simulink model "QiMotorController_ModelReference"  (R2021b)
settings: Solver=FixedStepDiscrete  StartTime=0.0  StopTime=5  RelTol=1e-3
PreLoadFcn:
  | RTWConfigurationCB('preloadfcn', bdroot);
PostLoadFcn:
  | load('configuration/data_struct.mat');
  | load('configuration/fluxMaps_propMotor.mat');
  | load('configuration/parameterInit_PROP.mat');
  | load('configuration/parameterInit_PUMP.mat');
  | load('configuration/parameterInit_PITCH.mat');
  | load('configuration/parameterInit_TILT.mat');
  | %load('configuration/base_workspace_signal_definition.mat');
  | %load('resolvedatastores_to_baseworkspace_for_faster_simulation.mat');
model workspace (MAT data in the model file):
  ADC_CALIBRATION_SAMPLES = Simulink.Parameter
  ADC_CALIBRATION_SAMPLES.Value = 20000
  ADC_CALIBRATION_SAMPLES.Description = 'Number of samples taken by the ADC offset/calibration 
    | function to calibrate the ADC values. Units are in number of 80kHz
    | control interrupts. The time taken to complete the calibration will be
    | equal to:
    | 
    | ADC_CALIBRATION_SAMPLES / (INVERTER_PWM_RATE * 2) seconds
    | '
  ADC_CALIBRATION_SAMPLES.DataType = 'uint32'
  ADC_CALIBRATION_SAMPLES.Complexity = 'real'
  ADC_CALIBRATION_SAMPLES.Dimensions = [1 1]
  DEFAULT_RESOLVER_CONTROL_WORD = Simulink.Parameter
  DEFAULT_RESOLVER_CONTROL_WORD.Value = 97
  DEFAULT_RESOLVER_CONTROL_WORD.DataType = 'uint32'
  DEFAULT_RESOLVER_CONTROL_WORD.Complexity = 'real'
  DEFAULT_RESOLVER_CONTROL_WORD.Dimensions = [1 1]
  PLL_FREQUENCY = Simulink.Parameter
  PLL_FREQUENCY.Value = 100000000
  PLL_FREQUENCY.Description = '100 MHz'
  PLL_FREQUENCY.DataType = 'double'
  PLL_FREQUENCY.Complexity = 'real'
  PLL_FREQUENCY.Dimensions = [1 1]
  SIMULATION_OPTIONS = Simulink.Parameter
  SIMULATION_OPTIONS.Value = 0
  SIMULATION_OPTIONS.Description = 'Set to ''0'' for normal Simulation
    | Set to ''1'' for "Flying Start" simulation'
  SIMULATION_OPTIONS.DataType = 'uint32'
  SIMULATION_OPTIONS.Complexity = 'real'
  SIMULATION_OPTIONS.Dimensions = [1 1]
  TARGET_CODE_GEN = Simulink.Parameter
  TARGET_CODE_GEN.Value = 0
  TARGET_CODE_GEN.Description = 'Set to ''0'' for Plant Model or PIL Simulation
    | Set to ''1'' for Target System Code Generation'
  TARGET_CODE_GEN.DataType = 'uint32'
  TARGET_CODE_GEN.Complexity = 'real'
  TARGET_CODE_GEN.Dimensions = [1 1]
  Ts = 2.5e-07
undefined symbols (not defined in the file): DEADTIME_NS__PITCH, DEADTIME_NS__PROP, DEADTIME_NS__PUMP, DEADTIME_NS__TILT, fIa_, fIb_, fIc_, fIdc_, fMotorEncoderFloat_, fMotorSensorSpeed_, fUa_, fUb_, fUc_, fUdc_, inbtilt, mdl_pitch_uiAPUFlags, mdl_pitch_uiFlags, modelData, oMot_, oOut_, opInputResolverData_, oPitch, oState_, PLANT_SPEED_QUADRATIC_COEFF__PUMP, POLE_PAIRS_INIT__PITCH, POLE_PAIRS_INIT__PROP, POLE_PAIRS_INIT__PUMP, POLE_PAIRS_INIT__TILT, PWM_FREQ_KHZ__PITCH, PWM_FREQ_KHZ__PROP, PWM_FREQ_KHZ__PUMP, R_PHASE_INIT__PITCH, R_PHASE_INIT__PROP, R_PHASE_INIT__TILT, R_PHASE_INIT_PLANT__PUMP, uiControlReadback_, uiGateDriverStatus_
libraries: simulink x51, spsSeriesRLCBranchLib x25, spsMosfetLib x24, powerlib_extras x24, spsCurrentMeasurementLib x17, spsVoltageMeasurementLib x17, spsPermanentMagnetSynchronousMachineLib x3, spsDCVoltageSourceLib x2, motorModelLibrary x2, slpidlib x2, cstblocks x1, spspowerguiLib x1
(part 1 of 5)
Description:
  | /************************************************************
  | /* (c) 2013 Phasor Systems, Incorporated
  | /* All rights reserved
  | /*
  | /* Model provided under End User License Agreement or OEM License Agreement
  | /*
  | /* Use of this model is your acceptance of the terms and conditions of these
  | /* agreements.
  | /*
  | /************************************************************
settings Model: ModifiedComment=Brad -- Sat Feb 01 15:53:39 2014 -- Version 1.11  Creator=Brad Landseadel  LastModifiedBy=jessica.colton
settings Model: ModifiedHistory=|
  | Brad -- Sat Feb 01 15:53:39 2014 -- Version 1.11
  | 
  | 
  | Brad -- Sat Feb 01 15:53:39 2014 -- Version 1.11
  | 
  | 
  | Brad -- Sat Feb 01 15:48:49 2014 -- Version 1.10
  | 
  | 
  | Brad -- Sat Feb 01 15:38:18 2014 -- Version 1.9
  | 
  | 
  | Brad -- Sat Feb 01 15:22:57 2014 -- Version 1.8
  | 
  | 
  | Brad -- Sat Feb 01 15:08:45 2014 -- Version 1.7
  | 
  | 
  | Brad -- Sat Feb 01 14:46:18 2014 -- Version 1.6
  | 
  | 
  | Brad -- Sat Feb 01 13:34:06 2014 -- Version 1.5
  | 
  | 
  | Brad -- Sat Feb 01 13:29:08 2014 -- Version 1.4
  | 
  | 
  | Brad -- Sat Feb 01 13:18:41 2014 -- Version 1.3
  | 
  | 
  | Brad -- Sat Feb 01 12:30:13 2014 -- Version 1.2
settings SolverCC: AlgebraicLoopSolver=TrustRegion  PositivePriorityOrder=on
settings DataIOCC: LimitDataPoints=on  SaveFormat=Array  SignalLoggingSaveFormat=ModelDataLogs  SaveOutput=off  SaveTime=off  ReturnWorkspaceOutputs=off
settings OptimizationCC: DefaultParameterBehavior=Inlined  GainParamInheritBuiltInType=on  UseFloatMulNetSlope=on  DefaultUnderspecifiedDataType=single  InlineInvariantSignals=on  StrengthReduction=on  PassReuseOutputArgsAs=Individual arguments  ExpressionDepthLimit=2147483647  ZeroExternalMemoryAtStartup=off  ZeroInternalMemoryAtStartup=off  NoFixptDivByZeroProtection=on  EfficientFloat2IntCast=on  MaxStackSize=2000  SimCompilerOptimization=on  AccelVerboseBuild=on  OptimizeBlockOrder=speed  UseRowMajorAlgorithm=on  OptimizationPriority=Speed  LabelGuidedReuse=on  MultiThreadedLoops=on  EfficientTunableParamExpr=on
settings DebuggingCC: ReadBeforeWriteMsg=DisableAll  WriteAfterReadMsg=DisableAll  MergeDetectMultiDrivingBlocksExec=none  SolverPrmCheckMsg=warning  MultiTaskDSMMsg=none  MultiTaskRateTransMsg=warning  ParameterTunabilityLossMsg=error  FixptConstUnderflowMsg=error  FixptConstOverflowMsg=error  BusObjectLabelMismatch=error  AssertControl=DisableAll  AllowSymbolicDim=off  StateNameClashWarn=warning  SFUnexpectedBacktrackingDiag=warning  SFNoUnconditionalDefaultTransitionDiag=warning  SFExecutionAtInitializationDiag=none  SFMachineParentedDataDiag=warning  ArithmeticOperatorsInVariantConditions=warning
settings HardwareCC: ProdBitPerPointer=32  ProdBitPerSizeT=32  ProdBitPerPtrDiffT=32  ProdLargestAtomicInteger=Long  ProdLargestAtomicFloat=Double  ProdWordSize=32  ProdHWDeviceType=ARM Compatible->ARM Cortex-A  TargetLargestAtomicInteger=Long  TargetLargestAtomicFloat=Double  TargetIntDivRoundTo=Zero  TargetEndianess=LittleEndian  TargetHWDeviceType=ARM Compatible->ARM Cortex-A
settings ModelReferenceCC: UpdateModelReferenceTargets=IfOutOfDate  PropagateSignalLabelsOutOfModel=off
settings SFSimCC: SimCustomHeaderCode="//#include \"custom_code/second_level_include/math_special.h\""  SimUserSources=//math_special.c  SimUserIncludeDirs=//custom_code/src/  SFSimEcho=off  SimUseLocalCustomCode=off  MATLABDynamicMemAlloc=off  CustomCodeUndefinedFunction=UseInterfaceOnly
settings RTWCC: Description=Embedded Coder  SystemTargetFile=ert.tlc  GenCodeOnly=on  PackageGeneratedCodeAndArtifacts=on  TemplateMakefile=ert_default_tmf  GenerateReport=on  RetainRTWFile=on  RTWUseLocalCustomCode=off  CustomSource=custom_code/src/math_special.c  Toolchain=GNU gcc/g++ | gmake (64-bit Linux)  BuildConfiguration=Faster Runs  IncludeHyperlinkInReport=on  LaunchReport=on  GenerateTraceInfo=on  GenerateTraceReport=on  GenerateTraceReportSl=on  GenerateTraceReportSf=on  GenerateTraceReportEml=on  GenerateWebview=on  GenerateCodeMetricsReport=on  GenerateCodeReplacementReport=on  CheckMdlBeforeBuild=Warning
settings RTWCC: CustomHeaderCode=|
  | #include "../custom_code/second_level_include/math_special.h"
  | 
  | // FPGA interface
  | #include "../custom_code/include/motorTask_int.h"
  | #include "../custom_code/include/motorControl_common.h"
  | #include "../custom_code/include/common.h"
  | #include "../custom_code/include/motorControl_adc.h"
  | #include "../custom_code/include/motorControl_pwm.h"
  | 
  | // InterCore
  | #include "../custom_code/inverter_shared_memory/legacy_inverter_shared_memory_declaration.h"
  | 
  | // Second Level Includes
  | #include "../custom_code/second_level_include/adc.h"
  | #include "../custom_code/second_level_include/application_layer_com.h"
  | #include "../custom_code/second_level_include/gate_enable.h"
  | #include "../custom_code/second_level_include/housekeeping.h"
  | #include "../custom_code/second_level_include/hw_defines.h"
  | #include "../custom_code/second_level_include/iir.h"
  | #include "../custom_code/second_level_include/legacy_interCoreCom.h"
  | #include "../custom_code/second_level_include/motor_control_main.h"
  | #include "../custom_code/second_level_include/motorControl_common.h"
  | #include "../custom_code/second_level_include/motorTask_init.h"
  | #include "../custom_code/second_level_include/motorTask_intercoreCom.h"
  | #include "../custom_code/second_level_include/motorTask_main.h"
  | #include "../custom_code/second_level_include/motorTask_StateMachine.h"
  | #include "../custom_code/second_level_include/parameter_init.h"
  | #include "../custom_code/second_level_include/pattern_generator.h"
  | #include "../custom_code/second_level_include/pi_controller.h"
  | #include "../custom_code/second_level_include/platform.h"
  | #include "../custom_code/second_level_include/pwm.h"
  | #include "../custom_code/second_level_include/resolver_driver.h"
  | #include "../custom_code/second_level_include/software_identity_data_storage.h"
  | #include "../custom_code/second_level_include/std_math.h"
settings CodeAppCC: ForceParamTrailComments=on  IgnoreCustomStorageClasses=off  IgnoreTestpoints=on  MaxIdLength=128  OperatorAnnotations=on  SimulinkDataObjDesc=on  SFDataObjDesc=on  InsertBlockDesc=on  StateflowObjectComments=on
settings ERTTargetCC: TargetLangStandard=C99 (ISO)  CombineSignalStateStructs=on  GroupInternalDataByFunction=on  SuppressErrorStatus=on  SupportComplex=off  ParenthesesLevel=Maximum  CastingMode=Explicit  RootIOFormat=Structure reference  ERTCustomFileTemplate=example_file_process.tlc
settings ConfigComp: CovMetricSettings=dw  CovSaveCumulativeToWorkspaceVar=on  CovSaveSingleToWorkspaceVar=on  CovExternalEMLEnable=off  CovSFcnEnable=off
settings SimscapeCC: SimscapeNormalizeSystem=off

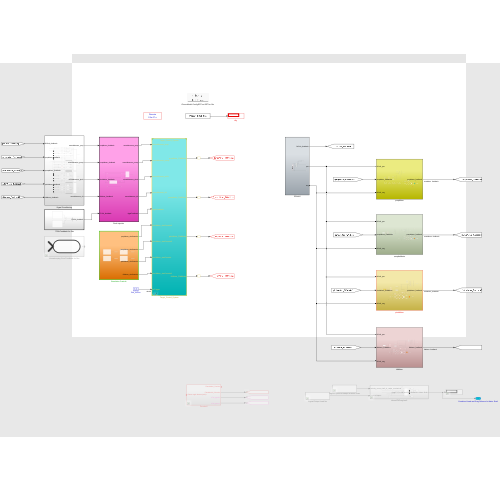
[thumbnail: Simulink's stored preview of the top-level diagram]
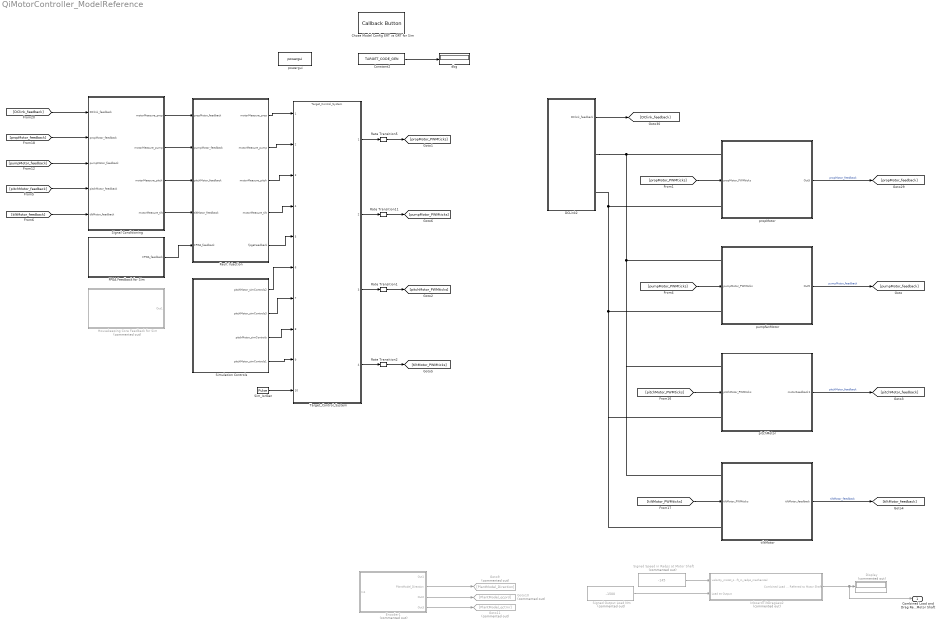
== system QiMotorController_ModelReference ==
  Chose Model Config ERT vs GRT for Sim : CallbackButton  ButtonText=Chose ERT vs GRT for Sim
      settings: ClickFcn=|
      | TARGET_CODE_GEN_LOCAL = getVariable( get_param('PMSM_Sensorless_Propulsion_Model_Code_Generation_Struct','ModelWorkspace'),'TARGET_CODE_GEN').Value;
      | 
      | if( TARGET_CODE_GEN_LOCAL == 0 )
      |  setActiveConfigSet('PMSM_Sensorless_Propulsion_Model_Code_Generation_Struct', 'grt_simulated_config');
      |  get_param(getActiveConfigSet('PMSM_Sensorless_Propulsion_Model_Code_Generation_Struct'),'Name')
      | end
      | 
      | if( TARGET_CODE_GEN_LOCAL == 1 )
      |  setActiveConfigSet('PMSM_Sensorless_Propulsion_Model_Code_Generation_Struct', 'Xilinx_Zynq_Core4');
      |  get_param(getActiveConfigSet('PMSM_Sensorless_Propulsion_Model_Code_Generation_Struct'),'Name')
      | end
  Constant2 : Constant  Value=TARGET_CODE_GEN  OutDataTypeStr=boolean  SampleTime=-1
  DCLink2 : Subsystem
  Display : Display  Commented=on
  Encoder1 : Subsystem  Commented=on
  FPGA Feedback for Sim : Subsystem  TreatAsAtomicUnit=on  SystemSampleTime=1/(PWM_FREQ_KHZ__PROP*1000)/2
  Fault Injection : Subsystem  TreatAsAtomicUnit=on  SystemSampleTime=1/(PWM_FREQ_KHZ__PROP*1000)/2
  Goto10 : Goto  Commented=on  GotoTag=PlantModel_qcprd
  Goto11 : Goto  Commented=on  GotoTag=PlantModel_qctmr
  Goto9 : Goto  Commented=on  GotoTag=PlantModel_Direction
  Housekeeping Core Feedback for Sim : Subsystem  Commented=on
  InboardTiltDragLaw2 : Subsystem  Commented=on
  Rate Transition{1..2,5,11} (4 alike) : RateTransition  Deterministic=off  OutPortSampleTime=Ts
  Signal Conditioning : Subsystem
  Signed Output Load Nm : Constant  Commented=on  Value=-1500  OutDataTypeStr=single  SampleTime=1e-2
  Signed Speed in Radps at Motor Shaft : Constant  Commented=on  Value=-145  OutDataTypeStr=single  SampleTime=1e-2
  Sim_IsrGen : DiscretePulseGenerator  PulseType=Time based  Period=1/(PWM_FREQ_KHZ__PROP*1000)/2  PulseWidth=50
  Simulation Controls : Subsystem  TreatAsAtomicUnit=on  SystemSampleTime=1/(PWM_FREQ_KHZ__PROP*1000)/2
  Target_Control_System : ModelReference  ModelNameDialog=Target_Control_System  SimulationMode=Normal  ModelReferenceVersion=4.101
  dbg : Display
      settings: Format=decimal (Stored Integer)
  pitchMotor : Subsystem
      settings: PortSchema="{\"entries\":[{\"content\":{\"sides\":[{\"content\":{\"connectorIds\":[\"LConn1\",\"In1\",\"LConn2\"]},\"type\":\"ConnectorPlacement.EquallySpacedRectSide\",\"uuid\":\"2948c356-2dfc-4425-a4d7-a3951926bd60\"},{\"content\":{\"connectorIds\":[\"Out1\"],\"side\":\"RIGHT\"},\"type\":\"ConnectorPlacement.EquallySpacedRectSide\",\"uuid\":\"906a8e9a-2635-4c14-9d40-34f0713bab39\"},{\"content\":{\"connectorIds\":[],\"side\":\"TOP\"},\"type\":\"ConnectorPlacement.EquallySpacedRectSide\",\"uuid\":\"336ec430-6931-46f0-bbde-94f235c37a61\"},{\"content\":{\"connectorIds\":[],\"side\":\"HIDDEN\"},\"type\":\"ConnectorPlacement.EquallySpacedRectSide\",\"uuid\":\"b760127f-7c64-4918-bd3a-cb813c8c851d\"}]},\"type\":\"ConnectorPlacement.EquallySpacedConnector\",\"uuid\":\"386eabba-acb8-4870-b3f4-1d48c2148e04\"}],\"packageUris\":[\"http://schema.mathworks.com/mf0/Connector/R2020b\"],\"version\":\"1.0\"}"
  powergui : spspowerguiLib/powergui  SimulationMode=Discrete  SampleTime=Ts  frequency=60  Iterations=50  frequencyindice=0  Pbase=100e6  ErrMax=1e-4  UnitsV=kV  UnitsW=MW  buscounter=0  FunctionMessages=off  echomessages=off  EnableUseOfTLC=off  CurrentSourceSwitches=off  DisableSnubberDevices=off  DisableRonSwitches=off  DisableVfSwitches=off  DisplayEquations=off  AutomaticDiscreteSolvers=off  SolverType=Tustin  Interpol=off  ExternalGateDelay=off  methode=off  Ts=0  x0status=blocks  SPID=off  SwTol=0  HookPort=off  NonlinearTolerance=1e-4  nMaxIteration=100  ContinueOnMaxIteration=off  RestoreLinks=warning  ResistiveCurrentMeasurement=off  Frange=[0:2:500]  Ylog=off  Xlog=on  ShowGrid=off  save=off  variable=ZData  structure=0  ZoomFFT=on  StartTime=0.0  cycles=1  DisplayStyle=1  fundamental=60  FreqAxis=off  MaxFrequency=1000  frequencyindicesteady=1  RmsSteady=1  display=off
  propMotor : Subsystem
      settings: PortSchema="{\"entries\":[{\"content\":{\"sides\":[{\"content\":{\"connectorIds\":[\"LConn1\",\"In1\",\"LConn2\"]},\"type\":\"ConnectorPlacement.EquallySpacedRectSide\",\"uuid\":\"2948c356-2dfc-4425-a4d7-a3951926bd60\"},{\"content\":{\"connectorIds\":[\"Out1\"],\"side\":\"RIGHT\"},\"type\":\"ConnectorPlacement.EquallySpacedRectSide\",\"uuid\":\"906a8e9a-2635-4c14-9d40-34f0713bab39\"},{\"content\":{\"connectorIds\":[],\"side\":\"TOP\"},\"type\":\"ConnectorPlacement.EquallySpacedRectSide\",\"uuid\":\"336ec430-6931-46f0-bbde-94f235c37a61\"},{\"content\":{\"connectorIds\":[],\"side\":\"HIDDEN\"},\"type\":\"ConnectorPlacement.EquallySpacedRectSide\",\"uuid\":\"b760127f-7c64-4918-bd3a-cb813c8c851d\"}]},\"type\":\"ConnectorPlacement.EquallySpacedConnector\",\"uuid\":\"386eabba-acb8-4870-b3f4-1d48c2148e04\"}],\"packageUris\":[\"http://schema.mathworks.com/mf0/Connector/R2020b\"],\"version\":\"1.0\"}"
  pumpfanMotor : Subsystem
      settings: PortSchema="{\"entries\":[{\"content\":{\"sides\":[{\"content\":{\"connectorIds\":[\"LConn1\",\"In1\",\"LConn2\"]},\"type\":\"ConnectorPlacement.EquallySpacedRectSide\",\"uuid\":\"2948c356-2dfc-4425-a4d7-a3951926bd60\"},{\"content\":{\"connectorIds\":[\"Out1\"],\"side\":\"RIGHT\"},\"type\":\"ConnectorPlacement.EquallySpacedRectSide\",\"uuid\":\"906a8e9a-2635-4c14-9d40-34f0713bab39\"},{\"content\":{\"connectorIds\":[],\"side\":\"TOP\"},\"type\":\"ConnectorPlacement.EquallySpacedRectSide\",\"uuid\":\"336ec430-6931-46f0-bbde-94f235c37a61\"},{\"content\":{\"connectorIds\":[],\"side\":\"HIDDEN\"},\"type\":\"ConnectorPlacement.EquallySpacedRectSide\",\"uuid\":\"b760127f-7c64-4918-bd3a-cb813c8c851d\"}]},\"type\":\"ConnectorPlacement.EquallySpacedConnector\",\"uuid\":\"386eabba-acb8-4870-b3f4-1d48c2148e04\"}],\"packageUris\":[\"http://schema.mathworks.com/mf0/Connector/R2020b\"],\"version\":\"1.0\"}"
  tiltMotor : Subsystem
      settings: PortSchema="{\"entries\":[{\"content\":{\"sides\":[{\"content\":{\"connectorIds\":[\"LConn1\",\"In1\",\"LConn2\"]},\"type\":\"ConnectorPlacement.EquallySpacedRectSide\",\"uuid\":\"2948c356-2dfc-4425-a4d7-a3951926bd60\"},{\"content\":{\"connectorIds\":[\"Out1\"],\"side\":\"RIGHT\"},\"type\":\"ConnectorPlacement.EquallySpacedRectSide\",\"uuid\":\"906a8e9a-2635-4c14-9d40-34f0713bab39\"},{\"content\":{\"connectorIds\":[],\"side\":\"TOP\"},\"type\":\"ConnectorPlacement.EquallySpacedRectSide\",\"uuid\":\"336ec430-6931-46f0-bbde-94f235c37a61\"},{\"content\":{\"connectorIds\":[],\"side\":\"HIDDEN\"},\"type\":\"ConnectorPlacement.EquallySpacedRectSide\",\"uuid\":\"b760127f-7c64-4918-bd3a-cb813c8c851d\"}]},\"type\":\"ConnectorPlacement.EquallySpacedConnector\",\"uuid\":\"386eabba-acb8-4870-b3f4-1d48c2148e04\"}],\"packageUris\":[\"http://schema.mathworks.com/mf0/Connector/R2020b\"],\"version\":\"1.0\"}"
  Combined Load and Drag Referred to Motor Shaft : Outport
  wires:
  Rate Transition5/1 -> [propMotor_PWMticks]
  Encoder1/2(PlantModel_Direction) -> Goto9/1
  Encoder1/3(Out2) -> Goto10/1
  Encoder1/4(Out3) -> Goto11/1
  Constant2/1 -> dbg/1
  [propMotor_PWMticks] -> propMotor/1(propMotor_PWMticks)
  DCLink2/1(DClink_feedback) -> [DClink_feedback]
  propMotor/1(Out5) -> [propMotor_feedback]  "propMotor_feedback"
  pumpfanMotor/1(Out5) -> [pumpMotor_feedback]  "pumpMotor_feedback"
  [pitchMotor_PWMticks] -> pitchMotor/1(pitchMotor_PWMticks)
  [tiltMotor_PWMticks] -> tiltMotor/1(tiltMotor_PWMticks)
  [pumpMotor_feedback] -> Signal Conditioning/3(pumpMotor_feedback)
  [propMotor_feedback] -> Signal Conditioning/2(propMotor_feedback)
  [DClink_feedback] -> Signal Conditioning/1(DClink_feedback)
  pitchMotor/1(motorFeedback1) -> [pitchMotor_feedback]  "pitchMotor_feedback"
  tiltMotor/1(tiltMotor_feedback) -> [tiltMotor_feedback]  "tiltMotor_feedback"
  [pumpMotor_PWMticks] -> pumpfanMotor/1(pumpMotor_PWMticks)
  [tiltMotor_feedback] -> Signal Conditioning/5(tiltMotor_feedback)
  [pitchMotor_feedback] -> Signal Conditioning/4(pitchMotor_feedback)
  Signal Conditioning/1(motorMeasure_prop) -> Fault Injection/1(propMotor_feedback)
  Signal Conditioning/2(motorMeasure_pump) -> Fault Injection/2(pumpMotor_feedback)
  Signal Conditioning/4(motorMeasure_tilt) -> Fault Injection/4(tiltMotor_feedback)
  Signal Conditioning/3(motorMeasure_pitch) -> Fault Injection/3(pitchMotor_feedback)
  Target_Control_System/2 -> Rate Transition11/1
  Rate Transition11/1 -> [pumpMotor_PWMticks]
  Target_Control_System/1 -> Rate Transition5/1
  Target_Control_System/3 -> Rate Transition1/1
  Rate Transition1/1 -> [pitchMotor_PWMticks]
  Signed Output Load Nm/1 -> InboardTiltDragLaw2/2(Load at Output)
  InboardTiltDragLaw2/1(Combined Load and Drag Referred to Motor Shaft) -> Display/1, Combined Load and Drag Referred to Motor Shaft/1
  Signed Speed in Radps at Motor Shaft/1 -> InboardTiltDragLaw2/1(velocity_motot_shaft_in_radps_mechanical)
  Rate Transition2/1 -> [tiltMotor_PWMticks]
  Target_Control_System/4 -> Rate Transition2/1
  FPGA Feedback for Sim/1(FPGA_feedback) -> Fault Injection/5(FPGA_feedback)
  Simulation Controls/1(pitchMotor_simControls2) -> Target_Control_System/6
  Simulation Controls/2(pitchMotor_simControls3) -> Target_Control_System/7
  Simulation Controls/3(pitchMotor_simControls) -> Target_Control_System/8
  Simulation Controls/4(pitchMotor_simControls1) -> Target_Control_System/9
  Fault Injection/1(motorMeasure_prop) -> Target_Control_System/1
  Fault Injection/5(fpgaFeedback) -> Target_Control_System/5
  Fault Injection/2(motorMeasure_pump) -> Target_Control_System/2
  Fault Injection/4(motorMeasure_tilt) -> Target_Control_System/4
  Fault Injection/3(motorMeasure_pitch) -> Target_Control_System/3
  Sim_IsrGen/1 -> Target_Control_System/10
  connections:
  DCLink2/RConn1 -- pitchMotor/LConn1 -- tiltMotor/LConn1 -- pumpfanMotor/LConn1 -- propMotor/LConn1
  tiltMotor/LConn2 -- pitchMotor/LConn2 -- pumpfanMotor/LConn2 -- DCLink2/RConn2 -- propMotor/LConn2

== system QiMotorController_ModelReference/DCLink2 ==
  Battery internal resistance2 : spsSeriesRLCBranchLib/Series RLC Branch  LConnTagsString=__new0  RConnTagsString=__new0  BranchType=R  Resistance=0.4  Inductance=33e-9  SetiL0=off  InitialCurrent=0  Capacitance=470e-6  Setx0=off  InitialVoltage=0  Measurements=None
  Bus Creator : BusCreator  Inputs=2
  CT2 : spsCurrentMeasurementLib/Current Measurement  PhasorSimulation=off  OutputType=Complex  PSBequivalent=0
  VDC4 : spsDCVoltageSourceLib/DC Voltage Source  Amplitude=700/2  Measurements=None
  VDC5 : spsDCVoltageSourceLib/DC Voltage Source  Amplitude=700/2  Measurements=None
  VM3 : spsVoltageMeasurementLib/Voltage Measurement  PhasorSimulation=off  OutputType=Complex  PSBequivalent=0
  pos : PMIOPort  Side=Right
  neg : PMIOPort  Port=2  Side=Right
  DClink_feedback : Outport
  wires:
  CT2/1 -> Bus Creator/1  "DClinkCurrent"
  Bus Creator/1 -> DClink_feedback/1  "DClink_feedback"
  VM3/1 -> Bus Creator/2  "DClinkVoltage"
  connections:
  VDC5/RConn1 -- Battery internal resistance2/RConn1
  VM3/LConn2 -- neg/RConn1 -- VDC4/LConn1
  CT2/RConn1 -- pos/RConn1
  VM3/LConn1 -- Battery internal resistance2/LConn1 -- CT2/LConn1
  VDC4/RConn1 -- VDC5/LConn1

== system QiMotorController_ModelReference/Encoder1 ==
  In1 : Inport
  1/T Simulation : Subsystem  Commented=on
  Convert rotor angle to counts : Constant  Value=2*pi/(4095*2)  SampleTime=-1
  Data Type Conversion : DataTypeConversion  OutDataTypeStr=uint16
  Detect Change : simulink/Logic and Bit Operations/Detect Change  Commented=on  vinit=0  OutDataTypeStr=boolean
  Detect Decrease : simulink/Logic and Bit Operations/Detect Decrease  vinit=0.0  OutDataTypeStr=boolean
  Detect Increase : simulink/Logic and Bit Operations/Detect Increase  vinit=0.0  OutDataTypeStr=boolean
  Display3 : Display
  Divide : Product  Inputs=*/  RndMeth=Nearest
  Goto6 : Goto  Commented=on  GotoTag=PM_eCAP_Capture
  Goto8 : Goto  Commented=on  GotoTag=PM_eCAP_TSCounter
  Logical Operator : Logic  IconShape=distinctive  AllPortsSameDT=off  OutDataTypeStr=boolean
  Logical Operator1 : Logic  Operator=NOT  IconShape=distinctive  AllPortsSameDT=off  OutDataTypeStr=boolean
  Math Function : Math  Operator=mod  SignedPower=on  SaturateOnIntegerOverflow=on
  Modulo : Constant  Value=4095*2  SampleTime=-1
  Scope2 : Scope  Commented=on  NumInputPorts=4
  Scope3 : Scope  Commented=on  NumInputPorts=3
  Unary Minus : UnaryMinus
  Out1 : Outport
  PlantModel_Direction : Outport  Port=2
  Out2 : Outport  Port=3
  Out3 : Outport  Port=4
  wires:
  Convert rotor angle to counts/1 -> Divide/2
  Divide/1 -> Math Function/1  "PlantModel_Position"
  Modulo/1 -> Math Function/2
  In1/1 -> Unary Minus/1
  Logical Operator/1 -> Scope2/3, PlantModel_Direction/1  "PlantModel_Direction"
  Detect Increase/1 -> Logical Operator/1
  Detect Decrease/1 -> Logical Operator1/1
  Logical Operator1/1 -> Logical Operator/2
  Unary Minus/1 -> Detect Decrease/1, Detect Increase/1, Scope2/1, Divide/1
  Math Function/1 -> Display3/1, Data Type Conversion/1
  1/T Simulation/1(Out1) -> Scope3/1, Goto6/1, Out2/1
  1/T Simulation/2(Out2) -> Out3/1, Goto8/1, Scope3/2
  Detect Change/1 -> 1/T Simulation/1(In3), Scope3/3
  Data Type Conversion/1 -> Scope2/2, Out1/1, Detect Change/1  "PlantModel_Position"

== system QiMotorController_ModelReference/FPGA Feedback for Sim ==
  Bus Creator2 : BusCreator  Inputs=2
  Rate Transition1 : RateTransition
  Rate Transition11 : RateTransition
  pitchMotor : Subsystem  TreatAsAtomicUnit=on
  tiltMotor : Subsystem  TreatAsAtomicUnit=on
  FPGA_feedback : Outport
  wires:
  pitchMotor/1(Out1) -> Rate Transition11/1  "pitchMotor_FPGAfeedback"
  Rate Transition1/1 -> Bus Creator2/2  "tiltMotor_FPGAfeedback"
  Rate Transition11/1 -> Bus Creator2/1  "pitchMotor_FPGAfeedback"
  tiltMotor/1(Out1) -> Rate Transition1/1  "tiltMotor_FPGAfeedback"
  Bus Creator2/1 -> FPGA_feedback/1

== system QiMotorController_ModelReference/Fault Injection ==
  propMotor_feedback : Inport  OutDataTypeStr=Bus: SAdcDataSingleIn_t
  pumpMotor_feedback : Inport  Port=2  OutDataTypeStr=Bus: SAdcDataSingleIn_t
  pitchMotor_feedback : Inport  Port=3  OutDataTypeStr=Bus: SAdcDataSingleIn_t
  tiltMotor_feedback : Inport  Port=4  OutDataTypeStr=Bus: SAdcDataSingleIn_t
  FPGA_feedback : Inport  Port=5
  Bus Assignment1 : BusAssignment  AssignedSignals=pitchMotor_FPGAfeedback
  Bus Selector : BusSelector  OutputSignals=pitchMotor_FPGAfeedback
  pitchMotor_faults : Subsystem  TreatAsAtomicUnit=on
  motorMeasure_prop : Outport  OutDataTypeStr=Bus: SAdcDataSingleIn_t
  motorMeasure_pump : Outport  Port=2  OutDataTypeStr=Bus: SAdcDataSingleIn_t
  motorMeasure_pitch : Outport  Port=3  OutDataTypeStr=Bus: SAdcDataSingleIn_t
  motorMeasure_tilt : Outport  Port=4  OutDataTypeStr=Bus: SAdcDataSingleIn_t
  fpgaFeedback : Outport  Port=5
  wires:
  propMotor_feedback/1 -> motorMeasure_prop/1
  pumpMotor_feedback/1 -> motorMeasure_pump/1
  tiltMotor_feedback/1 -> motorMeasure_tilt/1
  pitchMotor_feedback/1 -> pitchMotor_faults/1(pitchMotor_feedback)
  pitchMotor_faults/1(motorMeasure_pitch) -> motorMeasure_pitch/1
  FPGA_feedback/1 -> Bus Selector/1, Bus Assignment1/1
  pitchMotor_faults/2(fpgaFeedback_pitch) -> Bus Assignment1/2
  Bus Selector/1 -> pitchMotor_faults/2(pitchMotor_FPGAfeedback)  "<pitchMotor_FPGAfeedback>"
  Bus Assignment1/1 -> fpgaFeedback/1

== system QiMotorController_ModelReference/Housekeeping Core Feedback for Sim ==
  Out1 : Outport

== system QiMotorController_ModelReference/InboardTiltDragLaw2 ==
  velocity_motot_shaft_in_radps_mechanical : Inport
  Load at Output : Inport  Port=2
  DefaultTemp : Constant  Value=45  OutDataTypeStr=single  SampleTime=1e-2
  Display : Display
  Display1 : Display
  Display2 : Display
  DocBlock : simulink/Model-Wide Utilities/DocBlock  DocumentType=Text
      content=|
      | /// \breif Check in what drag mode we are currently running; this is for tilts only
      |    /// Logic table: -1, not floppy; -1 floppy;  use dMechanicalEfficiency_ in the 1st case; in the 2nd, does not matter FD does the calcs
      |    ///               0, not floppy;  0 floppy;  use dMechanicalEfficiency_ only for the 1st of the two
      |    ///               >0, not floppy; >0 floppy;  do not use dMechanicaEfficiency_ in either mode, i.e. set it to 1Type your documentation here
  DocBlock1 : simulink/Model-Wide Utilities/DocBlock  DocumentType=Text
      content=|
      | This is used to make comparison to stick torque when commensing actuator motion.
      | Defaulting to 0 for simplicity. Connect to actual electrical torque as needed for testing
  MotoredOrNot : Constant  OutDataTypeStr=single  SampleTime=1e-2
  SimplifiedVersion : Constant  Value=0  OutDataTypeStr=single  SampleTime=1e-2
  Subsystem1 : Subsystem
  Sum4 : Sum
  WhichDragCalcSeeDoc : Constant  OutDataTypeStr=single  SampleTime=1e-2
  drag2 : Subsystem
  Combined Load and Drag Referred to Motor Shaft : Outport
  wires:
  Subsystem1/1(torque_load_m) -> drag2/4(torque_load_m)
  velocity_motot_shaft_in_radps_mechanical/1 -> drag2/2(velocity_m)
  Sum4/1 -> Combined Load and Drag Referred to Motor Shaft/1, Display2/1
  WhichDragCalcSeeDoc/1 -> drag2/6(DrgMlt), Subsystem1/2(DrgMlt)
  DefaultTemp/1 -> drag2/3(motor_temp)
  SimplifiedVersion/1 -> drag2/1(torque_out_m)
  Load at Output/1 -> Subsystem1/1(torque_load)
  MotoredOrNot/1 -> drag2/5(n_invs), Subsystem1/3(n_inv)
  drag2/1(drag_torque) -> Display/1, Sum4/1
  drag2/2(load_torque) -> Sum4/2, Display1/1

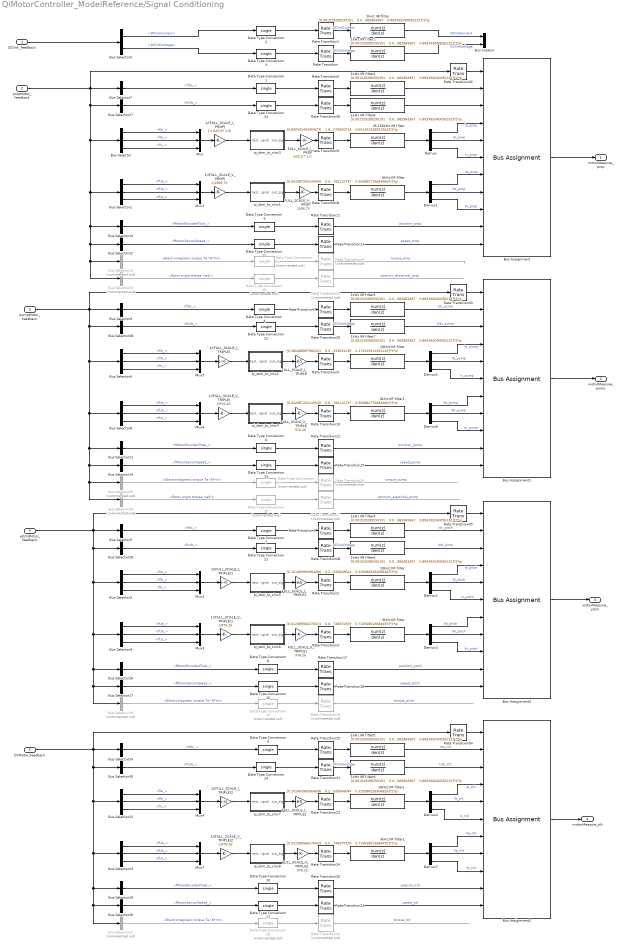
== system QiMotorController_ModelReference/Signal Conditioning ==
  DClink_feedback : Inport
  propMotor_feedback : Inport  Port=2  OutDataTypeStr=Bus: SAdcDataSingleIn_t
  pumpMotor_feedback : Inport  Port=3  OutDataTypeStr=Bus: SAdcDataSingleIn_t
  pitchMotor_feedback : Inport  Port=4  OutDataTypeStr=Bus: SAdcDataSingleIn_t
  tiltMotor_feedback : Inport  Port=5  OutDataTypeStr=Bus: SAdcDataSingleIn_t
  1/(FULL_SCALE_I_PROP) : Gain  Gain=1/(-625.0* 2.0)
  1/(FULL_SCALE_I_TRIPLE) : Gain  Gain=1/-65
  1/(FULL_SCALE_I_TRIPLE)1 : Gain  Gain=1/-65
  1/(FULL_SCALE_I_TRIPLE)2 : Gain  Gain=1/-65
  1/(FULL_SCALE_V_PROP) : Gain  Gain=1/1906.75
  1/(FULL_SCALE_V_TRIPLE) : Gain  Gain=1/976.26
  1/(FULL_SCALE_V_TRIPLE)1 : Gain  Gain=1/976.26
  1/(FULL_SCALE_V_TRIPLE)2 : Gain  Gain=1/976.26
  10kHz IIR filter : DiscreteFilter  Numerator="[0.101483969364696    0.202967938729392    0.101483969364696]*2*pi"  Denominator="[1.0000   -0.919150650848044    0.325086528306828]*2*pi"
  10kHz IIR filter1 : DiscreteFilter  Numerator="[0.101483969364696    0.202967938729392    0.101483969364696]*2*pi"  Denominator="[1.0000   -0.919150650848044    0.325086528306828]*2*pi"
  19kHz IIR filter : DiscreteFilter  Numerator="[0.280488997983221    0.560977995966443    0.280488997983221]*2*pi"  Denominator="[1.0000   -0.050059919631235    0.172015911564120]*2*pi"
  1kHz IIR filter{,1..9} (10 alike) : DiscreteFilter  Numerator="[0.001529289293191    0.003058578586383    0.001529289293191]*2*pi"  Denominator="[1.0000   -1.886374882883367    0.892492040056132]*2*pi"
  35.156kHz IIR filter : DiscreteFilter  Numerator="[0.800592403464570    1.601184806929140    0.800592403464570]*2*pi"  Denominator="[1.0000   1.561018075800718    0.641351538057563]*2*pi"
  3kHz IIR filter : DiscreteFilter  Numerator="[0.012389566278474    0.024779132556948    0.012389566278474]*2*pi"  Denominator="[1.0000   -1.661369748570559    0.710928013684455]*2*pi"
  3kHz IIR filter1 : DiscreteFilter  Numerator="[0.012389566278474    0.024779132556948    0.012389566278474]*2*pi"  Denominator="[1.0000   -1.661369748570559    0.710928013684455]*2*pi"
  6kHz IIR filter : DiscreteFilter  Numerator="[0.042987254143545    0.085974508287089    0.042987254143545]*2*pi"  Denominator="[1.0000   -1.333933760110787    0.505882776684966]*2*pi"
  6kHz IIR filter1 : DiscreteFilter  Numerator="[0.042987254143545    0.085974508287089    0.042987254143545]*2*pi"  Denominator="[1.0000   -1.333933760110787    0.505882776684966]*2*pi"
  Bus Assignment{,1..3} (4 alike) : BusAssignment  AssignedSignals=fIdc_,fUdc_,fIa_,fIb_,fIc_,fUa_,fUb_,fUc_,fMotorEncoderFloat_,fMotorSensorSpeed_
  Bus Creator : BusCreator  Inputs=2
  Bus Selector{,3,6,22} (4 alike) : BusSelector  OutputSignals=fIa_,fIb_,fIc_
  Bus Selector{1,4,8,23} (4 alike) : BusSelector  OutputSignals=fUa_,fUb_,fUc_
  Bus Selector{10..11,16,19} (4 alike) : BusSelector  OutputSignals=fMotorEncoderFloat_
  Bus Selector{12,14,17,20} (4 alike) : BusSelector  OutputSignals=fMotorSensorSpeed_
  Bus Selector{13,15,18,21} (4 alike) : BusSelector  Commented=on  OutputSignals=Electromagnetic torque Te (N*m)
  Bus Selector2 : BusSelector  OutputSignals=DClinkCurrent,DClinkVoltage
  Bus Selector{5,7,9,24} (4 alike) : BusSelector  OutputSignals=fIdc_
  Bus Selector25 : BusSelector  Commented=on  OutputSignals=Rotor angle thetae (rad)
  Bus Selector26 : BusSelector  Commented=on  OutputSignals=Rotor angle thetae (rad)
  Bus Selector{27..30} (4 alike) : BusSelector  OutputSignals=fUdc_
  Data Type Conversion{1..11,13,15,17,21..24} (18 alike) : DataTypeConversion  OutDataTypeStr=single
  Data Type Conversion{12,14,16,18..20} (6 alike) : DataTypeConversion  Commented=on  OutDataTypeStr=single
  Demux{,1..7} (8 alike) : Demux  Outputs=3
  FULL_SCALE_I_PROP : Gain  Gain=-625.0 * 2.0
  FULL_SCALE_I_TRIPLE : Gain  Gain=-65
  FULL_SCALE_I_TRIPLE1 : Gain  Gain=-65
  FULL_SCALE_I_TRIPLE2 : Gain  Gain=-65
  FULL_SCALE_V_PROP : Gain  Gain=1906.75
  FULL_SCALE_V_TRIPLE : Gain  Gain=976.26
  FULL_SCALE_V_TRIPLE1 : Gain  Gain=976.26
  FULL_SCALE_V_TRIPLE2 : Gain  Gain=976.26
  Mux{,1..7} (8 alike) : Mux  Inputs=3
  Rate Transition{,28..31} (5 alike) : RateTransition  InitialCondition=700  OutPortSampleTime=1/(PWM_FREQ_KHZ__PROP*1000)*0.5
  Rate Transition{1..13,15,17..18,20..21,23..25,32..35} (25 alike) : RateTransition  OutPortSampleTime=1/(PWM_FREQ_KHZ__PROP*1000)*0.5
  Rate Transition{14,16,19,22,26..27} (6 alike) : RateTransition  Commented=on  OutPortSampleTime=1/(PWM_FREQ_KHZ__PROP*1000)*0.5
  qi_dsm_to_sinc1 : Subsystem
  qi_dsm_to_sinc2 : Subsystem
  qi_dsm_to_sinc3 : Subsystem
  qi_dsm_to_sinc4 : Subsystem
  qi_dsm_to_sinc5 : Subsystem
  qi_dsm_to_sinc6 : Subsystem
  qi_dsm_to_sinc7 : Subsystem
  qi_dsm_to_sinc8 : Subsystem
  motorMeasure_prop : Outport  OutDataTypeStr=Bus: SAdcDataSingleIn_t
  motorMeasure_pump : Outport  Port=2  OutDataTypeStr=Bus: SAdcDataSingleIn_t
  motorMeasure_pitch : Outport  Port=3  OutDataTypeStr=Bus: SAdcDataSingleIn_t
  motorMeasure_tilt : Outport  Port=4  OutDataTypeStr=Bus: SAdcDataSingleIn_t
  wires:
  propMotor_feedback/1 -> Rate Transition32/1, Bus Selector25/1, Bus Selector13/1, Bus Selector12/1, Bus Selector10/1, Bus Selector1/1, Bus Selector/1, Bus Selector27/1, Bus Selector7/1
  Bus Selector/2 -> Mux/2  "<fIb_>"
  Bus Selector/1 -> Mux/1  "<fIa_>"
  Bus Selector/3 -> Mux/3  "<fIc_>"
  Mux/1 -> 1/(FULL_SCALE_I_PROP)/1
  Bus Selector1/1 -> Mux1/1  "<fUa_>"
  Bus Selector1/2 -> Mux1/2  "<fUb_>"
  Bus Selector1/3 -> Mux1/3  "<fUc_>"
  Mux1/1 -> 1/(FULL_SCALE_V_PROP)/1
  6kHz IIR filter/1 -> Demux1/1
  Bus Selector2/1 -> Data Type Conversion2/1  "<DClinkCurrent>"
  Bus Selector2/2 -> Data Type Conversion3/1  "<DClinkVoltage>"
  DClink_feedback/1 -> Bus Selector2/1
  Demux/1 -> Bus Assignment/4  "Ia_prop"
  Demux/2 -> Bus Assignment/5  "Ib_prop"
  Demux/3 -> Bus Assignment/6  "Ic_prop"
  Demux1/1 -> Bus Assignment/7  "Va_prop"
  Demux1/2 -> Bus Assignment/8  "Vb_prop"
  Demux1/3 -> Bus Assignment/9  "Vc_prop"
  Bus Selector3/1 -> Mux2/1  "<fIa_>"
  Bus Selector3/2 -> Mux2/2  "<fIb_>"
  Bus Selector3/3 -> Mux2/3  "<fIc_>"
  Bus Selector4/1 -> Mux3/1  "<fUa_>"
  Bus Selector4/2 -> Mux3/2  "<fUb_>"
  Bus Selector4/3 -> Mux3/3  "<fUc_>"
  Mux3/1 -> 1/(FULL_SCALE_V_TRIPLE)1/1
  Demux2/1 -> Bus Assignment3/4  "Ia_pitch"
  Demux2/2 -> Bus Assignment3/5  "Ib_pitch"
  Demux2/3 -> Bus Assignment3/6  "Ic_pitch"
  Demux3/1 -> Bus Assignment3/7  "Va_pitch"
  Demux3/2 -> Bus Assignment3/8  "Vb_pitch"
  Demux3/3 -> Bus Assignment3/9  "Vc_pitch"
  Rate Transition9/1 -> 35.156kHz IIR filter/1
  35.156kHz IIR filter/1 -> Demux/1
  Demux5/1 -> Bus Assignment1/4  "Ia_pump"
  Rate Transition5/1 -> 19kHz IIR filter/1
  Demux5/3 -> Bus Assignment1/6  "Ic_pump"
  Bus Selector6/1 -> Mux5/1  "<fIa_>"
  19kHz IIR filter/1 -> Demux5/1
  Demux5/2 -> Bus Assignment1/5  "Ib_pump"
  Bus Selector6/2 -> Mux5/2  "<fIb_>"
  Bus Selector6/3 -> Mux5/3  "<fIc_>"
  Data Type Conversion1/1 -> Rate Transition6/1
  1kHz IIR filter2/1 -> Bus Assignment/2
  Rate Transition6/1 -> 1kHz IIR filter2/1
  Bus Selector7/1 -> Data Type Conversion1/1  "<fIdc_>"
  1kHz IIR filter1/1 -> Bus Creator/2  "DClinkVoltage"
  Rate Transition/1 -> 1kHz IIR filter1/1  "DClinkVoltage"
  Data Type Conversion3/1 -> Rate Transition/1
  Rate Transition1/1 -> 1kHz IIR filter/1  "DClinkCurrent"
  Data Type Conversion2/1 -> Rate Transition1/1
  1kHz IIR filter/1 -> Bus Creator/1  "DClinkCurrent"
  Demux6/3 -> Bus Assignment1/9  "Vc_pump"
  Bus Selector8/2 -> Mux6/2  "<fUb_>"
  Bus Selector8/3 -> Mux6/3  "<fUc_>"
  Demux6/1 -> Bus Assignment1/7  "Va_pump"
  Bus Selector8/1 -> Mux6/1  "<fUa_>"
  Demux6/2 -> Bus Assignment1/8  "Vb_pump"
  Rate Transition10/1 -> 6kHz IIR filter1/1
  6kHz IIR filter1/1 -> Demux6/1
  qi_dsm_to_sinc1/1(out_sig) -> FULL_SCALE_V_PROP/1
  Rate Transition8/1 -> 6kHz IIR filter/1
  Rate Transition7/1 -> 1kHz IIR filter3/1
  Data Type Conversion4/1 -> Rate Transition7/1
  Bus Selector9/1 -> Data Type Conversion4/1  "<fIdc_>"
  1kHz IIR filter3/1 -> Bus Assignment1/2  "Idc_pump"
  Data Type Conversion5/1 -> Rate Transition11/1
  Bus Selector10/1 -> Data Type Conversion5/1  "<fMotorEncoderFloat_>"
  Rate Transition11/1 -> Bus Assignment/10  "position_prop"
  Bus Selector11/1 -> Data Type Conversion6/1  "<fMotorEncoderFloat_>"
  Data Type Conversion6/1 -> Rate Transition12/1
  Rate Transition12/1 -> Bus Assignment1/10  "position_pump"
  Bus Selector12/1 -> Data Type Conversion11/1  "<fMotorSensorSpeed_>"
  Bus Selector13/1 -> Data Type Conversion12/1  "<Electromagnetic torque Te (N*m)>"
  Rate Transition13/1 -> Bus Assignment/11  "speed_prop"
  Rate Transition14/1 -> ?  "torque_prop"
  Bus Selector15/1 -> Data Type Conversion14/1  "<Electromagnetic torque Te (N*m)>"
  Bus Selector14/1 -> Data Type Conversion13/1  "<fMotorSensorSpeed_>"
  pumpMotor_feedback/1 -> Bus Selector28/1, Bus Selector11/1, Bus Selector14/1, Bus Selector26/1, Bus Selector15/1, Bus Selector8/1, Bus Selector6/1, Rate Transition33/1, Bus Selector9/1
  Rate Transition16/1 -> ?  "torque_pump"
  Rate Transition15/1 -> Bus Assignment1/11  "speed_pump"
  1kHz IIR filter4/1 -> Bus Assignment3/2  "Idc_pitch"
  Bus Selector5/1 -> Data Type Conversion7/1  "<fIdc_>"
  Rate Transition4/1 -> 1kHz IIR filter4/1
  Data Type Conversion7/1 -> Rate Transition4/1
  3kHz IIR filter/1 -> Demux3/1
  Rate Transition3/1 -> 3kHz IIR filter/1
  qi_dsm_to_sinc6/1(out_sig) -> FULL_SCALE_V_TRIPLE1/1
  Rate Transition19/1 -> ?  "torque_pitch"
  Rate Transition18/1 -> Bus Assignment3/11  "speed_pitch"
  Bus Selector16/1 -> Data Type Conversion8/1  "<fMotorEncoderFloat_>"
  Data Type Conversion8/1 -> Rate Transition17/1
  Bus Selector18/1 -> Data Type Conversion16/1  "<Electromagnetic torque Te (N*m)>"
  Bus Selector17/1 -> Data Type Conversion15/1  "<fMotorSensorSpeed_>"
  Rate Transition17/1 -> Bus Assignment3/10  "position_pitch"
  Bus Selector20/1 -> Data Type Conversion17/1  "<fMotorSensorSpeed_>"
  1kHz IIR filter5/1 -> Bus Assignment2/2  "Idc_tilt"
  Bus Selector22/2 -> Mux4/2  "<fIb_>"
  Bus Selector23/1 -> Mux7/1  "<fUa_>"
  Rate Transition24/1 -> 3kHz IIR filter1/1
  Mux4/1 -> 1/(FULL_SCALE_I_TRIPLE)2/1
  Demux4/1 -> Bus Assignment2/4  "Ia_tilt"
  Bus Selector24/1 -> Data Type Conversion9/1  "<fIdc_>"
  Mux7/1 -> 1/(FULL_SCALE_V_TRIPLE)2/1
  Demux7/2 -> Bus Assignment2/8  "Vb_tilt"
  Data Type Conversion9/1 -> Rate Transition25/1
  Bus Selector23/3 -> Mux7/3  "<fUc_>"
  Demux7/3 -> Bus Assignment2/9  "Vc_tilt"
  Bus Selector22/1 -> Mux4/1  "<fIa_>"
  Demux4/3 -> Bus Assignment2/6  "Ic_tilt"
  Bus Selector22/3 -> Mux4/3  "<fIc_>"
  Rate Transition22/1 -> ?  "torque_tilt"
  qi_dsm_to_sinc8/1(out_sig) -> FULL_SCALE_V_TRIPLE2/1
  Rate Transition25/1 -> 1kHz IIR filter5/1
  Bus Selector23/2 -> Mux7/2  "<fUb_>"
  10kHz IIR filter1/1 -> Demux4/1
  Bus Selector19/1 -> Data Type Conversion10/1  "<fMotorEncoderFloat_>"
  Rate Transition23/1 -> 10kHz IIR filter1/1
  Rate Transition20/1 -> Bus Assignment2/10  "position_tilt"
  Bus Selector21/1 -> Data Type Conversion18/1  "<Electromagnetic torque Te (N*m)>"
  Demux4/2 -> Bus Assignment2/5  "Ib_tilt"
  Demux7/1 -> Bus Assignment2/7  "Va_tilt"
  3kHz IIR filter1/1 -> Demux7/1
  Rate Transition21/1 -> Bus Assignment2/11  "speed_tilt"
  10kHz IIR filter/1 -> Demux2/1
  qi_dsm_to_sinc3/1(out_sig) -> FULL_SCALE_I_PROP/1
  Data Type Conversion11/1 -> Rate Transition13/1
  Data Type Conversion12/1 -> Rate Transition14/1
  Data Type Conversion13/1 -> Rate Transition15/1
  Data Type Conversion14/1 -> Rate Transition16/1
  qi_dsm_to_sinc5/1(out_sig) -> FULL_SCALE_I_TRIPLE1/1
  Mux2/1 -> 1/(FULL_SCALE_I_TRIPLE)1/1
  Rate Transition2/1 -> 10kHz IIR filter/1
  Data Type Conversion15/1 -> Rate Transition18/1
  Data Type Conversion16/1 -> Rate Transition19/1
  Data Type Conversion17/1 -> Rate Transition21/1
  Data Type Conversion18/1 -> Rate Transition22/1
  1/(FULL_SCALE_I_PROP)/1 -> qi_dsm_to_sinc3/1(test_signal)
  1/(FULL_SCALE_V_PROP)/1 -> qi_dsm_to_sinc1/1(test_signal)
  FULL_SCALE_I_PROP/1 -> Rate Transition9/1
  FULL_SCALE_V_PROP/1 -> Rate Transition8/1
  Mux6/1 -> 1/(FULL_SCALE_V_TRIPLE)/1
  1/(FULL_SCALE_V_TRIPLE)/1 -> qi_dsm_to_sinc4/1(test_signal)
  qi_dsm_to_sinc4/1(out_sig) -> FULL_SCALE_V_TRIPLE/1
  FULL_SCALE_V_TRIPLE/1 -> Rate Transition10/1
  Mux5/1 -> 1/(FULL_SCALE_I_TRIPLE)/1
  1/(FULL_SCALE_I_TRIPLE)/1 -> qi_dsm_to_sinc2/1(test_signal)
  qi_dsm_to_sinc2/1(out_sig) -> FULL_SCALE_I_TRIPLE/1
  FULL_SCALE_I_TRIPLE/1 -> Rate Transition5/1
  1/(FULL_SCALE_I_TRIPLE)1/1 -> qi_dsm_to_sinc5/1(test_signal)
  FULL_SCALE_I_TRIPLE1/1 -> Rate Transition2/1
  1/(FULL_SCALE_V_TRIPLE)1/1 -> qi_dsm_to_sinc6/1(test_signal)
  FULL_SCALE_V_TRIPLE1/1 -> Rate Transition3/1
  1/(FULL_SCALE_I_TRIPLE)2/1 -> qi_dsm_to_sinc7/1(test_signal)
  qi_dsm_to_sinc7/1(out_sig) -> FULL_SCALE_I_TRIPLE2/1
  FULL_SCALE_I_TRIPLE2/1 -> Rate Transition23/1
  Data Type Conversion10/1 -> Rate Transition20/1
  1/(FULL_SCALE_V_TRIPLE)2/1 -> qi_dsm_to_sinc8/1(test_signal)
  FULL_SCALE_V_TRIPLE2/1 -> Rate Transition24/1
  Bus Selector25/1 -> Data Type Conversion19/1  "<Rotor angle thetae (rad)>"
  Data Type Conversion19/1 -> Rate Transition26/1
  Rate Transition26/1 -> ?  "position_electrical_prop"
  Rate Transition27/1 -> ?  "position_electrical_pump"
  Data Type Conversion20/1 -> Rate Transition27/1
  Bus Selector26/1 -> Data Type Conversion20/1  "<Rotor angle thetae (rad)>"
  Data Type Conversion23/1 -> Rate Transition30/1
  1kHz IIR filter8/1 -> Bus Assignment/3
  Rate Transition30/1 -> 1kHz IIR filter8/1
  Bus Selector27/1 -> Data Type Conversion23/1  "<fUdc_>"
  Data Type Conversion22/1 -> Rate Transition29/1
  1kHz IIR filter7/1 -> Bus Assignment1/3  "Udc_pump"
  Rate Transition29/1 -> 1kHz IIR filter7/1  "DClinkVoltage"
  Bus Selector28/1 -> Data Type Conversion22/1  "<fUdc_>"
  pitchMotor_feedback/1 -> Bus Selector29/1, Bus Selector4/1, Bus Selector16/1, Bus Selector17/1, Bus Selector18/1, Bus Selector3/1, Rate Transition35/1, Bus Selector5/1
  Data Type Conversion21/1 -> Rate Transition28/1
  Bus Selector29/1 -> Data Type Conversion21/1  "<fUdc_>"
  1kHz IIR filter6/1 -> Bus Assignment3/3  "Udc_pitch"
  Rate Transition28/1 -> 1kHz IIR filter6/1  "DClinkVoltage"
  tiltMotor_feedback/1 -> Rate Transition34/1, Bus Selector30/1, Bus Selector22/1, Bus Selector23/1, Bus Selector21/1, Bus Selector20/1, Bus Selector19/1, Bus Selector24/1
  Data Type Conversion24/1 -> Rate Transition31/1
  1kHz IIR filter9/1 -> Bus Assignment2/3  "Udc_tilt"
  Bus Selector30/1 -> Data Type Conversion24/1  "<fUdc_>"
  Rate Transition31/1 -> 1kHz IIR filter9/1  "DClinkVoltage"
  Bus Assignment/1 -> motorMeasure_prop/1
  Rate Transition32/1 -> Bus Assignment/1
  Bus Assignment1/1 -> motorMeasure_pump/1
  Rate Transition33/1 -> Bus Assignment1/1
  Rate Transition34/1 -> Bus Assignment2/1
  Bus Assignment2/1 -> motorMeasure_tilt/1
  Bus Assignment3/1 -> motorMeasure_pitch/1
  Rate Transition35/1 -> Bus Assignment3/1

== system QiMotorController_ModelReference/Simulation Controls ==
  pitchMotor : Subsystem
  propMotor : Subsystem
  pumpMotor : Subsystem
  tiltMotor : Subsystem
  pitchMotor_simControls2 : Outport
  pitchMotor_simControls3 : Outport  Port=2
  pitchMotor_simControls : Outport  Port=3
  pitchMotor_simControls1 : Outport  Port=4
  wires:
  tiltMotor/1(Out1) -> pitchMotor_simControls1/1  "tiltMotor_simControls"
  pumpMotor/1(Out1) -> pitchMotor_simControls3/1  "pumpMotor_simControls"
  propMotor/1(Out1) -> pitchMotor_simControls2/1  "propMotor_simControls"
  pitchMotor/1(Out1) -> pitchMotor_simControls/1  "pitchMotor_simControls"

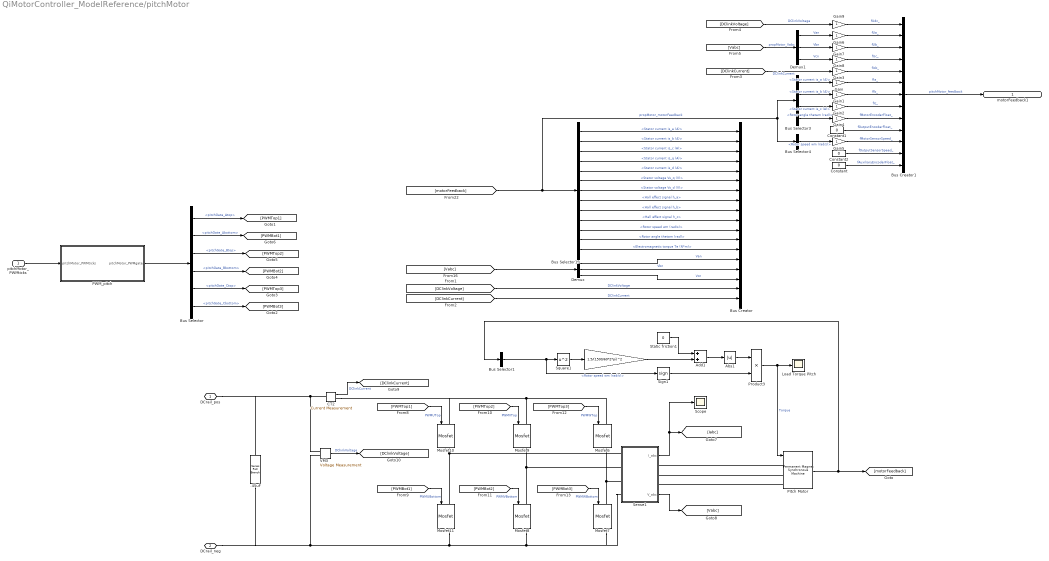
== system QiMotorController_ModelReference/pitchMotor ==
  pitchMotor_PWMticks : Inport
  " " : Gain  Gain=1.5/(1500/60*2*pi)^2
  .45uF : spsSeriesRLCBranchLib/Series RLC Branch  LConnTagsString=__new0  RConnTagsString=__new0  BranchType=C  Resistance=1  Inductance=1e-3  SetiL0=off  InitialCurrent=0  Capacitance=.45e-6  Setx0=off  InitialVoltage=0  Measurements=Branch voltage and current
  Abs1 : Abs
  Add1 : Sum
  Bus Creator : BusCreator  Inputs=18
  Bus Creator1 : BusCreator  Inputs=13  OutDataTypeStr=Bus: SAdcDataSingleIn_t
  Bus Selector : BusSelector  OutputSignals=pitchGate_Atop,pitchGate_Abottom,pitchGate_Btop,pitchGate_Bbottom,pitchGate_Ctop,pitchGate_Cbottom
  Bus Selector1 : BusSelector  OutputSignals=Rotor speed wm (rad/s)
  Bus Selector15 : BusSelector  OutputSignals=Stator current is_a (A),Stator current is_b (A),Stator current is_c (A),Stator current is_q (A),Stator current is_d (A),Stator voltage Vs_q (V),Stator voltage Vs_d (V),Hall effect signal h_a,Hall effect signal h_b,Hall effect signal h_c,Rotor speed wm (rad/s),Rotor angle thetam (rad),Electromagnetic torque Te (N*m)
  Bus Selector3 : BusSelector  OutputSignals=Stator current is_a (A),Stator current is_b (A),Stator current is_c (A),Rotor angle thetam (rad)
  Bus Selector4 : BusSelector  OutputSignals=Rotor speed wm (rad/s)
  CT2 : spsCurrentMeasurementLib/Current Measurement  PhasorSimulation=off  OutputType=Complex  PSBequivalent=0
  Constant : Constant  Value=0  OutDataTypeStr=single
  Constant1 : Constant  Value=0  OutDataTypeStr=single
  Constant2 : Constant  Value=0  OutDataTypeStr=single
  Demux : Demux  Outputs=3
  Demux1 : Demux  Outputs=3
  Gain{,1..9} (10 alike) : Gain  OutDataTypeStr=single
  Load Torque Pitch : Scope
  Mosfet{6..11} (6 alike) : spsMosfetLib/Mosfet  Ron=5e-3  Lon=0  Rd=0.01  Vfd=0  IC=0  Rs=1e5  Cs=inf  Measurements=on
  PWM_pitch : Subsystem
  Pitch Motor : spsPermanentMagnetSynchronousMachineLib/Permanent Magnet Synchronous Machine  NbPhases=3  FluxDistribution=Sinusoidal  RotorType=Round  MechanicalLoad=Torque Tm  PresetModel=No  ShowDetailedParameters=on  MeasurementBus=off  Resistance=R_PHASE_INIT__PITCH  Inductance=0  dqInductances=[160e-6 130e-6]  La=LS_INIT__PITCH  MachineConstant=Torque Constant (N.m / A_peak)  Flux=0.070667  VoltageCst=128.1752  TorqueCst=TORQUE_NM_PER_AMP_INIT__PITCH  Flat=0  Mechanical=[0.001 0.005 POLE_PAIRS_INIT__PITCH]  PolePairs=POLE_PAIRS_INIT__PROP  InitialConditions=[0,0,0,0]  InitialConditions5ph=[0 0 0 0 0 0]  RefAngle=Aligned with phase A axis (original Park)  IterativeDiscreteModel=Trapezoidal non iterative  TsBlock=Ts  TsPowergui=0
      link override From: GotoTag=tp8169b85b_15ba_4846_bb0f_92caecca5899
      settings: AttributesFormatString=\n
  Product3 : Product
  Scope : Scope
  Sense1 : Subsystem
      settings: PortSchema="{\"entries\":[{\"content\":{\"sides\":[{\"content\":{\"connectorIds\":[\"LConn1\",\"LConn2\",\"LConn3\",\"LConn4\"]},\"type\":\"ConnectorPlacement.EquallySpacedRectSide\",\"uuid\":\"7842130e-3042-4aab-b72e-eb1cdec29ee8\"},{\"content\":{\"connectorIds\":[\"Out1\",\"RConn1\",\"RConn2\",\"RConn3\",\"Out2\"],\"side\":\"RIGHT\"},\"type\":\"ConnectorPlacement.EquallySpacedRectSide\",\"uuid\":\"c17ee381-f168-491a-818a-60a0284cb5f0\"},{\"content\":{\"connectorIds\":[],\"side\":\"TOP\"},\"type\":\"ConnectorPlacement.EquallySpacedRectSide\",\"uuid\":\"c745f3af-6fcc-4aa3-a9ef-8419a9649519\"}]},\"type\":\"ConnectorPlacement.EquallySpacedConnector\",\"uuid\":\"04fba2a7-cbbf-4a24-95eb-69eefae2f6e3\"}],\"packageUris\":[\"http://schema.mathworks.com/mf0/Connector/R2020b\"],\"version\":\"1.0\"}"
  Sign1 : Signum
  Square1 : Math  Operator=square  SaturateOnIntegerOverflow=on
  Static friction1 : Constant  Value=0  SampleTime=-1
  VM3 : spsVoltageMeasurementLib/Voltage Measurement  PhasorSimulation=off  OutputType=Complex  PSBequivalent=0
  DCrail_pos : PMIOPort  Side=Left
  DCrail_neg : PMIOPort  Port=2  Side=Left
  motorFeedback1 : Outport  OutDataTypeStr=Bus: SAdcDataSingleIn_t
  wires:
  [PWMTop2] -> Mosfet9/1  "PWMVTop"
  [PWMBot3] -> Mosfet7/1  "PWMWBottom"
  Sense1/2(V_abc) -> [Vabc]
  [PWMBot1] -> Mosfet11/1  "PWMUBottom"
  [PWMTop1] -> Mosfet10/1  "PWMUTop"
  [PWMTop3] -> Mosfet6/1  "PWMWTop"
  Sense1/1(I_abc) -> Scope/1, [Iabc]
  [PWMBot2] -> Mosfet8/1  "PWMVBottom"
  Bus Selector/3 -> [PWMTop2]  "<pitchGate_Btop>"
  Bus Selector/1 -> [PWMTop1]  "<pitchGate_Atop>"
  Bus Selector/2 -> [PWMBot1]  "<pitchGate_Abottom>"
  Bus Selector/4 -> [PWMBot2]  "<pitchGate_Bbottom>"
  Bus Selector/6 -> [PWMBot3]  "<pitchGate_Cbottom>"
  Bus Selector/5 -> [PWMTop3]  "<pitchGate_Ctop>"
  Demux/3 -> Bus Creator/16  "Vcn"
  Bus Selector15/2 -> Bus Creator/2  "<Stator current is_b (A)>"
  Demux/1 -> Bus Creator/14  "Van"
  Demux/2 -> Bus Creator/15  "Vbn"
  Bus Selector15/12 -> Bus Creator/12  "<Rotor angle thetam (rad)>"
  Bus Selector15/13 -> Bus Creator/13  "<Electromagnetic torque Te (N*m)>"
  Bus Selector15/10 -> Bus Creator/10  "<Hall effect signal h_c>"
  Bus Selector15/8 -> Bus Creator/8  "<Hall effect signal h_a>"
  Bus Selector15/3 -> Bus Creator/3  "<Stator current is_c (A)>"
  Bus Selector15/11 -> Bus Creator/11  "<Rotor speed wm (rad/s)>"
  Bus Selector15/4 -> Bus Creator/4  "<Stator current is_q (A)>"
  Bus Selector15/6 -> Bus Creator/6  "<Stator voltage Vs_q (V)>"
  Bus Selector15/9 -> Bus Creator/9  "<Hall effect signal h_b>"
  Bus Selector15/5 -> Bus Creator/5  "<Stator current is_d (A)>"
  Bus Selector15/1 -> Bus Creator/1  "<Stator current is_a (A)>"
  Bus Selector15/7 -> Bus Creator/7  "<Stator voltage Vs_d (V)>"
  [Vabc] -> Demux/1
  PWM_pitch/1(pitchMotor_PWMgates) -> Bus Selector/1
  pitchMotor_PWMticks/1 -> PWM_pitch/1(pitchMotor_PWMticks)
  CT2/1 -> [DClinkCurrent]  "DClinkCurrent"
  VM3/1 -> [DClinkVoltage]  "DClinkVoltage"
  [DClinkCurrent] -> Bus Creator/18  "DClinkCurrent"
  [DClinkVoltage] -> Bus Creator/17  "DClinkVoltage"
  Product3/1 -> Pitch Motor/1, Load Torque Pitch/1  "Torque"
  Add1/1 -> Abs1/1
  Static friction1/1 -> Add1/1
  Square1/1 -> " "/1
  " "/1 -> Add1/2
  Abs1/1 -> Product3/1
  Bus Selector1/1 -> Sign1/1, Square1/1  "<Rotor speed wm (rad/s)>"
  Pitch Motor/1 -> Bus Selector1/1, [motorFeedback]
  Sign1/1 -> Product3/2
  Bus Creator1/1 -> motorFeedback1/1  "pitchMotor_feedback"
  Gain3/1 -> Bus Creator1/5  "fIdc_"
  Demux1/2 -> Gain7/1  "Vbn"
  Bus Selector4/1 -> Gain5/1  "<Rotor speed wm (rad/s)>"
  Bus Selector3/2 -> Gain1/1  "<Stator current is_b (A)>"
  Gain9/1 -> Bus Creator1/1  "fUdc_"
  Constant2/1 -> Bus Creator1/12  "fOutputSensorSpeed_"
  Bus Selector3/4 -> Gain4/1  "<Rotor angle thetam (rad)>"
  Bus Selector3/3 -> Gain2/1  "<Stator current is_c (A)>"
  Gain4/1 -> Bus Creator1/9  "fMotorEncoderFloat_"
  Gain8/1 -> Bus Creator1/4  "fUc_"
  Gain5/1 -> Bus Creator1/11  "fMotorSensorSpeed_"
  Gain2/1 -> Bus Creator1/8  "fIc_"
  Gain/1 -> Bus Creator1/6  "fIa_"
  Gain7/1 -> Bus Creator1/3  "fUb_"
  Constant1/1 -> Bus Creator1/10  "fOutputEncoderFloat_"
  Constant/1 -> Bus Creator1/13  "fAuxiliaryEncoderFloat_"
  Demux1/3 -> Gain8/1  "Vcn"
  Bus Selector3/1 -> Gain/1  "<Stator current is_a (A)>"
  Demux1/1 -> Gain6/1  "Van"
  Gain1/1 -> Bus Creator1/7  "fIb_"
  [Vabc] -> Demux1/1  "propMotor_Vabc"
  [DClinkVoltage] -> Gain9/1  "DClinkVoltage"
  [DClinkCurrent] -> Gain3/1  "DClinkCurrent"
  Gain6/1 -> Bus Creator1/2  "fUa_"
  [motorFeedback] -> Bus Selector3/1, Bus Selector4/1, Bus Selector15/1  "propMotor_motorFeedback"
  connections:
  Mosfet6/LConn1 -- Mosfet10/LConn1 -- CT2/RConn1 -- Mosfet9/LConn1
  Mosfet11/RConn1 -- .45uF/RConn1 -- DCrail_neg/RConn1 -- VM3/LConn2 -- Mosfet8/RConn1 -- Mosfet7/RConn1 -- Sense1/LConn4
  Mosfet7/LConn1 -- Sense1/LConn3 -- Mosfet6/RConn1
  Mosfet8/LConn1 -- Sense1/LConn2 -- Mosfet9/RConn1
  Mosfet11/LConn1 -- Sense1/LConn1 -- Mosfet10/RConn1
  Pitch Motor/LConn1 -- Sense1/RConn1
  Pitch Motor/LConn2 -- Sense1/RConn2
  Pitch Motor/LConn3 -- Sense1/RConn3
  CT2/LConn1 -- .45uF/LConn1 -- DCrail_pos/RConn1 -- VM3/LConn1
